simulink model "statefdbk_integral_real"  (R2023b)
settings: Solver=ode45  StartTime=0.0  StopTime=20  RelTol=1e-3
values from neighbouring files (symbols this model uses):
  A = [A zeros(n,1); -C_ 1]    [control_integral.m]    (also in model.mat = [2.19826062055 1 0 0 0 0 -0.950981109251 0 1 0 0 0 ... (36 e; square_2V_2_5hz_100fs.mat = [3.68944323306 1 0 0 0 0 0 0 0 0 0 -4.87835143564 ... (121 e; square_2V_2_5hz_50fs.mat = [3.32314178319 1 0 0 0 0 0 0 0 0 0 -4.05203564565 ... (121 e)
  B = [B ; 0]    [control_integral.m]    (also in model.mat = [1 0 0 0 0 0]; square_2V_2_5hz_100fs.mat = [1 0 0 0 0 0 0 0 0 0 0]; square_2V_2_5hz_50fs.mat = [1 0 0 0 0 0 0 0 0 0 0])
  C_ = C    [control.m]    (also in control_integral.m)
  K = dlqr(A,B,Q,R)    [control.m]    (also in control_integral.m = K(1:end-1))
  Ki = K(end)    [control_integral.m]
  L = dlqe(A,G,C,Q_w,R_v)    [control.m]    (also in control_integral.m; plotter.m = convlength(L,'in','m')*100)
undefined symbols (not defined in the file or in its folder): MIO, National_Instruments, PCI
libraries: sldrtlib x3
settings Model: Creator=Tiago  LastModifiedBy=tiago
settings SolverCC: AlgebraicLoopSolver=TrustRegion
settings DataIOCC: ReturnWorkspaceOutputs=off
settings OptimizationCC: LifeSpan=inf
settings DebuggingCC: UnconnectedInputMsg=warning  UnconnectedOutputMsg=warning  UnconnectedLineMsg=warning  SFExecutionAtInitializationDiag=none  ArithmeticOperatorsInVariantConditions=warning
settings HardwareCC: ProdBitPerSizeT=32  ProdBitPerPtrDiffT=32  ProdWordSize=32  ProdHWDeviceType=Specified
settings SFSimCC: CustomCodeUndefinedFunction=UseInterfaceOnly
settings CodeAppCC: StateflowObjectComments=on

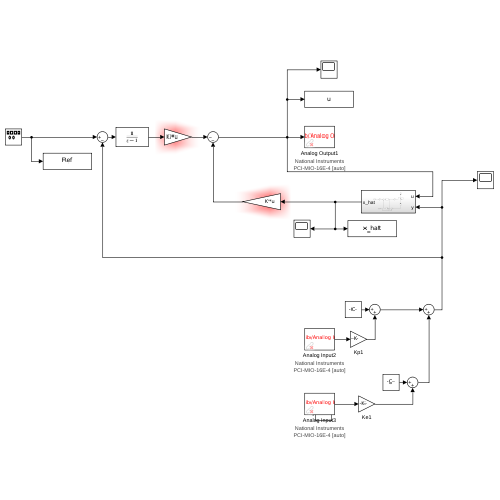
[thumbnail: Simulink's stored preview of the top-level diagram]
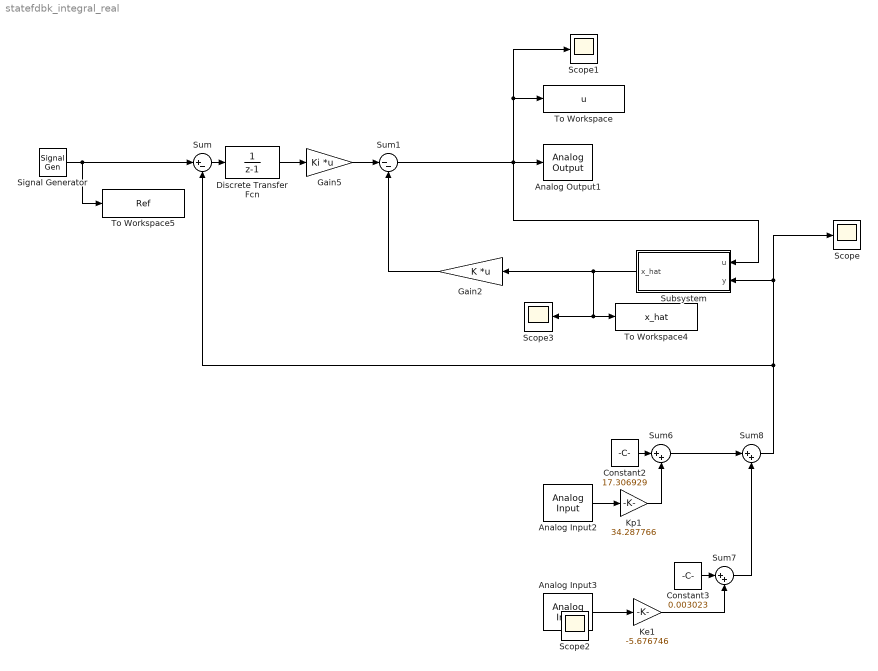
== system statefdbk_integral_real ==
  Analog Input2 : sldrtlib/Analog Input  SampleTime=0.02  MaxMissedTicks=10  ShowMissedTicks=off  YieldWhenWaiting=off  DrvName=National_Instruments/PCI-MIO-16E-4  DrvAddress=4294967295  DrvOptions=[0 0 0 0 0 0]  Channels=1  RangeMode=1  VoltRange=1  DataType=1
      settings: AttributesFormatString=National Instruments\nPCI-MIO-16E-4 [auto]
  Analog Input3 : sldrtlib/Analog Input  SampleTime=0.02  MaxMissedTicks=10  ShowMissedTicks=off  YieldWhenWaiting=off  DrvName=National_Instruments/PCI-MIO-16E-4  DrvAddress=4294967295  DrvOptions=[0 0 0 0 0 0]  Channels=2  RangeMode=1  VoltRange=1  DataType=1
      settings: AttributesFormatString=National Instruments\nPCI-MIO-16E-4 [auto]
  Analog Output1 : sldrtlib/Analog Output  SampleTime=0.02  MaxMissedTicks=10  ShowMissedTicks=off  YieldWhenWaiting=off  DrvName=National_Instruments/PCI-MIO-16E-4  DrvAddress=4294967295  DrvOptions=[0 0 0 0 0 0]  Channels=1  RangeMode=1  VoltRange=1  InitialValue=0  FinalValue=0
      settings: AttributesFormatString=National Instruments\nPCI-MIO-16E-4 [auto]
  Constant2 : Constant  Value=17.306929
  Constant3 : Constant  Value=0.003023
  Discrete Transfer Fcn : DiscreteTransferFcn  Denominator=[1 -1]
  Gain2 : Gain  Gain=K  Multiplication=Matrix(K*u)
  Gain5 : Gain  Gain=Ki  Multiplication=Matrix(K*u)
  Ke1 : Gain  Gain=-5.676746
  Kp1 : Gain  Gain=34.287766
  Scope{,1..3} (4 alike) : Scope
  Signal Generator : SignalGenerator  WaveForm=square  Amplitude=20  Frequency=0.5
  Subsystem : Subsystem
  Sum : Sum  Inputs=|+-
  Sum1 : Sum  Inputs=|--
  Sum6 : Sum  Inputs=|++
  Sum7 : Sum  Inputs=|++
  Sum8 : Sum  Inputs=|++
  To Workspace : ToWorkspace  VariableName=u  SaveFormat=Structure With Time  SampleTime=0.02
  To Workspace4 : ToWorkspace  VariableName=x_hat  SaveFormat=Structure With Time  SampleTime=0.02
  To Workspace5 : ToWorkspace  VariableName=Ref  SaveFormat=Structure With Time  SampleTime=-1
  wires:
  Subsystem/1(x_hat) -> Scope3/1, To Workspace4/1, Gain2/1
  Signal Generator/1 -> Sum/1, To Workspace5/1
  Sum1/1 -> Analog Output1/1, Subsystem/1(u), Scope1/1, To Workspace/1
  Gain2/1 -> Sum1/2
  Gain5/1 -> Sum1/1
  Sum/1 -> Discrete Transfer Fcn/1
  Discrete Transfer Fcn/1 -> Gain5/1
  Analog Input2/1 -> Kp1/1
  Ke1/1 -> Sum7/2
  Sum6/1 -> Sum8/1
  Constant2/1 -> Sum6/1
  Constant3/1 -> Sum7/1
  Analog Input3/1 -> Ke1/1
  Kp1/1 -> Sum6/2
  Sum7/1 -> Sum8/2
  Sum8/1 -> Sum/2, Scope/1, Subsystem/2(y)

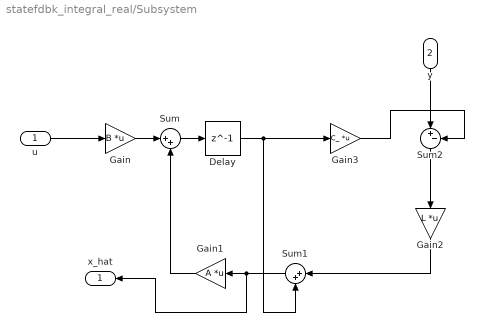
== system statefdbk_integral_real/Subsystem ==
  u : Inport
  y : Inport  Port=2
  Delay : Delay  DelayLength=1  InitialCondition=0
  Gain : Gain  Gain=B  Multiplication=Matrix(K*u)
  Gain1 : Gain  Gain=A  Multiplication=Matrix(K*u)
  Gain2 : Gain  Gain=L  Multiplication=Matrix(K*u)
  Gain3 : Gain  Gain=C_  Multiplication=Matrix(K*u)
  Sum : Sum  Inputs=|++
  Sum1 : Sum  Inputs=|++
  Sum2 : Sum  Inputs=|+-
  x_hat : Outport
  wires:
  u/1 -> Gain/1
  Gain3/1 -> Sum2/2
  y/1 -> Sum2/1
  Sum2/1 -> Gain2/1
  Gain2/1 -> Sum1/1
  Delay/1 -> Gain3/1, Sum1/2
  Sum1/1 -> x_hat/1, Gain1/1
  Gain/1 -> Sum/1
  Sum/1 -> Delay/1
  Gain1/1 -> Sum/2
